simulink model "test"  (R2016b)
settings: Solver=FixedStepAuto  StartTime=0.0  StopTime=Inf  FixedStep=0.01  RelTol=1e-3
undefined symbols (not defined in the file or in its folder): Angular, Linear
libraries: robotlib x3, simulink x3
settings Model: Creator=labpc  LastModifiedBy=labpc

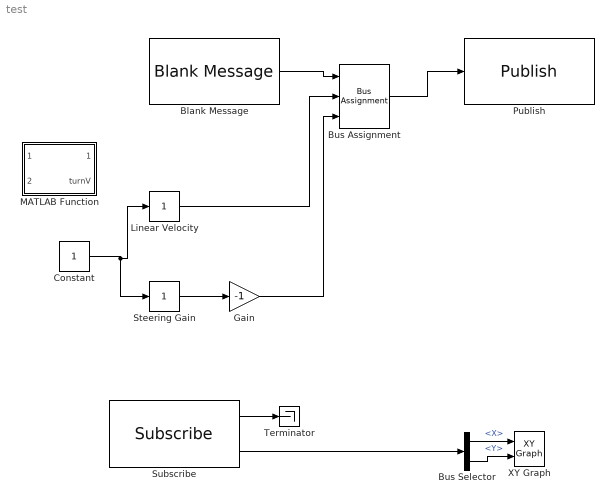
== system test ==
  Blank Message : robotlib/Blank Message  SourceLibraryInfo=This block requires Robotics System Toolbox  messageType=geometry_msgs/Twist  SampleTime=inf
  Bus Assignment : BusAssignment  AssignedSignals=Linear.X,Angular.Z
  Bus Selector : BusSelector  OutputSignals=Pose.Pose.Position.X,Pose.Pose.Position.Y
  Constant : Constant
  Gain : Gain  Gain=-1
  Linear Velocity : simulink/Math Operations/Slider Gain  low=0  gain=1  high=2
  MATLAB Function : MATLAB Function  TreatAsAtomicUnit=on
  Publish : robotlib/Publish  SourceLibraryInfo=This block requires Robotics System Toolbox  topicSource=Select from ROS network  topic=/mobile_base/commands/velocity  messageType=geometry_msgs/Twist  messageQueueLength=1
  Steering Gain : simulink/Math Operations/Slider Gain  low=-1  gain=1  high=1
  Subscribe : robotlib/Subscribe  SourceLibraryInfo=This block requires Robotics System Toolbox  topicSource=Select from ROS network  topic=/odom  messageType=nav_msgs/Odometry  sampleTime=-1  messageQueueLength=1
  Terminator : Terminator
  XY Graph : simulink/Sinks/XY Graph  xmin=-1  xmax=1  ymin=-1  ymax=1  st=-1
  wires:
  Blank Message/1 -> Bus Assignment/1
  Bus Assignment/1 -> Publish/1
  Constant/1 -> Linear Velocity/1, Steering Gain/1
  Steering Gain/1 -> Gain/1
  Linear Velocity/1 -> Bus Assignment/2
  Gain/1 -> Bus Assignment/3
  Subscribe/2 -> Bus Selector/1
  Bus Selector/1 -> XY Graph/1  "<X>"
  Bus Selector/2 -> XY Graph/2  "<Y>"
  Subscribe/1 -> Terminator/1

== matlab function test/MATLAB Function ==
  data: forwardVel input; turnVel input; forwardV output; turnV output
function [forwardV, turnV] = TurtleBotKeyboardTeleop(forwardVel,turnVel)
    
    % Modified MATLAB example code to publish only velocity messages and
    % nothing else. 

%     persistent velMsg

    
    keyObj = ExampleHelperTurtleBotKeyInput();
    
    disp('Keyboard Control: ');
    disp('i=forward, k=backward, j=left, l=right');
    disp('q=quit');
    disp('Waiting for input: ');
    
    % Use ASCII key representations for reply, initialize here
    reply = 0;
 
    while reply~='q'
         
        forwardV = 0;   % Initialize linear and angular velocities
        turnV = 0;
        
        reply = getKeystroke(keyObj);
        switch reply
            case 'i'         % i
                forwardV = forwardVel;
            case 'k'     % k
                forwardV = -forwardVel;
            case 'j'     % j
                turnV = turnVel;
            case 'l'     % l
                turnV = -turnVel;
        end
% 
%         if isempty(velMsg)
%             velMsg = rosmessage(velPub);
%         end
% 
%         velMsg.Linear.X = forwardV;
%         velMsg.Angular.Z = turnV;
% 
%         send(velPub,velMsg);

        pause(0.1);
    
    end
     
    closeFigure(keyObj);
    
end
